simulink model "test_motor"  (R2019a)
settings: Solver=VariableStepAuto  StartTime=0.0  StopTime=0.25  RelTol=1e-3
settings Model: Creator=abhis  LastModifiedBy=abhis

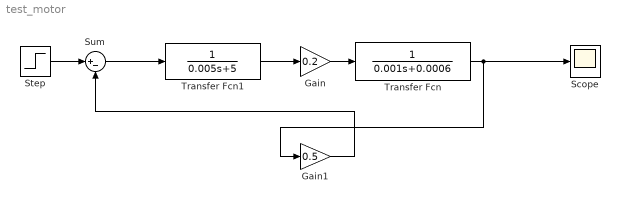
== system test_motor ==
  Gain : Gain  Gain=0.2
  Gain1 : Gain  Gain=0.5
  Scope : Scope
  Step : Step  Time=0  After=10  SampleTime=0
  Sum : Sum  Inputs=|+-
  Transfer Fcn : TransferFcn  Denominator=[0.001 0.0006]
  Transfer Fcn1 : TransferFcn  Denominator=[0.005 5]
  wires:
  Transfer Fcn1/1 -> Gain/1
  Gain/1 -> Transfer Fcn/1
  Gain1/1 -> Sum/2
  Transfer Fcn/1 -> Gain1/1, Scope/1
  Step/1 -> Sum/1
  Sum/1 -> Transfer Fcn1/1
